simulink model "Prova_es1_sim"  (R2022b)
settings: Solver=VariableStepAuto  StartTime=0.0  StopTime=10.0  RelTol=1e-3
undefined symbols (not defined in the file or in its folder): den, Kd, Ki, Kp, Kw, num, Tl
settings Model: Creator=marcoverri  LastModifiedBy=emanuelevitetta

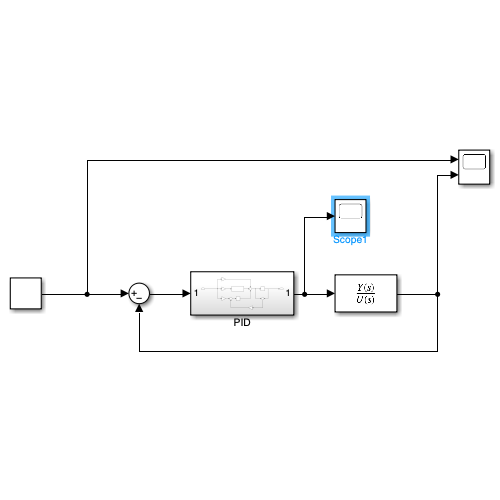
[thumbnail: Simulink's stored preview of the top-level diagram]
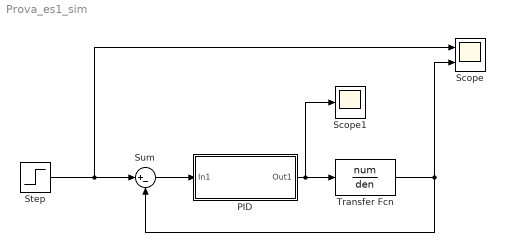
== system Prova_es1_sim ==
  PID : Subsystem
  Scope : Scope  NumInputPorts=2
  Scope1 : Scope
  Step : Step  After=10  SampleTime=0
  Sum : Sum  Inputs=|+-
  Transfer Fcn : TransferFcn  Numerator=num  Denominator=den
  wires:
  Step/1 -> Scope/1, Sum/1
  Sum/1 -> PID/1(In1)
  PID/1(Out1) -> Scope1/1, Transfer Fcn/1
  Transfer Fcn/1 -> Sum/2, Scope/2

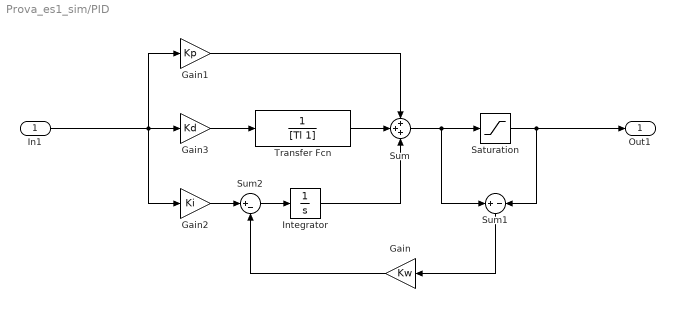
== system Prova_es1_sim/PID ==
  In1 : Inport
  Gain : Gain  Gain=Kw
  Gain1 : Gain  Gain=Kp
  Gain2 : Gain  Gain=Ki
  Gain3 : Gain  Gain=Kd
  Integrator : Integrator
  Saturation : Saturate  UpperLimit=10  LowerLimit=-10
  Sum : Sum  Inputs=+++
  Sum1 : Sum  Inputs=+-
  Sum2 : Sum  Inputs=|+-
  Transfer Fcn : TransferFcn  Numerator=[0 1]  Denominator=[Tl 1]
  Out1 : Outport
  wires:
  Gain1/1 -> Sum/1
  Gain3/1 -> Transfer Fcn/1
  In1/1 -> Gain2/1, Gain3/1, Gain1/1
  Sum/1 -> Sum1/1, Saturation/1
  Saturation/1 -> Out1/1, Sum1/2
  Gain2/1 -> Sum2/1
  Sum2/1 -> Integrator/1
  Sum1/1 -> Gain/1
  Transfer Fcn/1 -> Sum/2
  Integrator/1 -> Sum/3
  Gain/1 -> Sum2/2
